simulink library "magField_lib"  (R2018b)
settings: Solver=VariableStepAuto  StartTime=0.0  StopTime=10.0  RelTol=1e-3
undefined symbols (not defined in the file or in its folder): Earth, fswParams, WGS84
libraries: aerolibtransform2 x3, aerolibgravity2 x1
settings Model: Creator=Kate  LastModifiedBy=devantormey

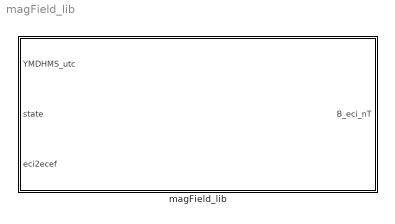
== system magField_lib ==
  magField_lib : Subsystem

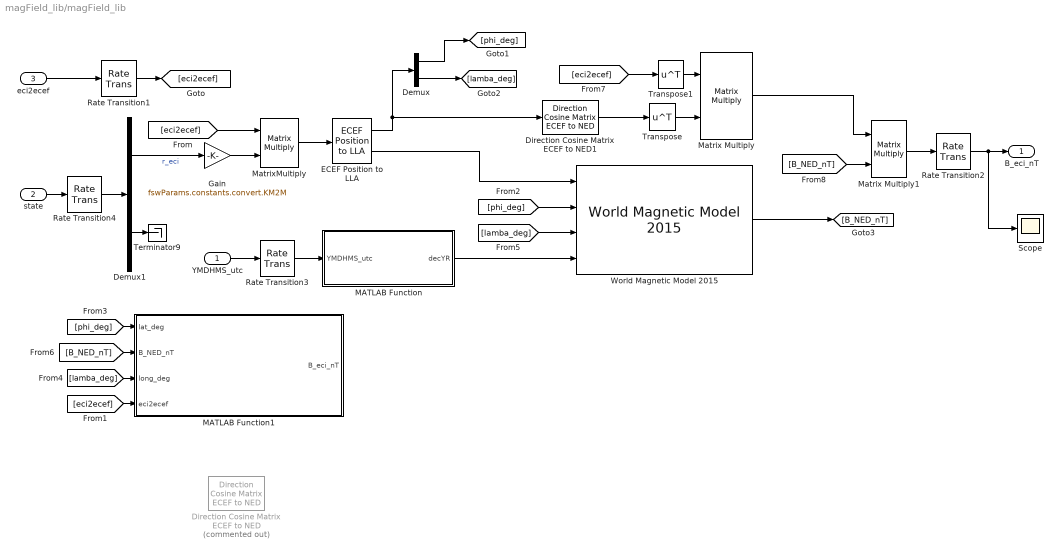
== system magField_lib/magField_lib ==
  YMDHMS_utc : Inport
  state : Inport  Port=2
  eci2ecef : Inport  Port=3
  Demux : Demux  Outputs=[1 1]
  Demux1 : Demux  Outputs=[3 10]
  Direction Cosine Matrix ECEF to NED : aerolibtransform2/Direction Cosine Matrix ECEF to NED  Commented=on
      settings: SourceProductName=Aerospace Blockset  SourceProductBaseCode=AE
  Direction Cosine Matrix ECEF to NED1 : aerolibtransform2/Direction Cosine Matrix ECEF to NED
      settings: SourceProductName=Aerospace Blockset  SourceProductBaseCode=AE
  ECEF Position to LLA : aerolibtransform2/ECEF Position to LLA  units=Metric (MKS)  ptype=Earth (WGS84)  F=1/298.257223563  R=6378137
      settings: SourceProductName=Aerospace Blockset  SourceProductBaseCode=AE
  Gain : Gain  Gain=fswParams.constants.convert.KM2M
  MATLAB Function : MATLAB Function  TreatAsAtomicUnit=on
  MATLAB Function1 : MATLAB Function  TreatAsAtomicUnit=on
  Matrix Multiply : Product  Multiplication=Matrix(*)
  Matrix Multiply1 : Product  Multiplication=Matrix(*)
  MatrixMultiply : Product  Multiplication=Matrix(*)
  Rate Transition1 : RateTransition  OutPortSampleTime=simParams.magField.sample_time_s
  Rate Transition2 : RateTransition
  Rate Transition3 : RateTransition  OutPortSampleTime=simParams.magField.sample_time_s
  Rate Transition4 : RateTransition  OutPortSampleTime=simParams.magField.sample_time_s
  Scope : Scope
  Terminator9 : Terminator
  Transpose : Math  Operator=transpose  SaturateOnIntegerOverflow=on
  Transpose1 : Math  Operator=transpose  SaturateOnIntegerOverflow=on
  World Magnetic Model 2015 : aerolibgravity2/World Magnetic Model 2015  units=Metric (MKS)  time_in=on  month=January  day=1  year=2015  action=Error  h_out=off  dec_out=off  inc_out=off  ti_out=off
      settings: SourceProductName=Aerospace Blockset  SourceProductBaseCode=AE
  B_eci_nT : Outport
  wires:
  Gain/1 -> MatrixMultiply/2
  Matrix Multiply1/1 -> Rate Transition2/1
  Rate Transition2/1 -> B_eci_nT/1, Scope/1
  [B_NED_nT] -> Matrix Multiply1/2
  Matrix Multiply/1 -> Matrix Multiply1/1
  Transpose/1 -> Matrix Multiply/2
  Transpose1/1 -> Matrix Multiply/1
  [eci2ecef] -> Transpose1/1
  Direction Cosine Matrix ECEF to NED1/1 -> Transpose/1
  Demux/2 -> [lamba_deg]
  Demux/1 -> [phi_deg]
  ECEF Position to LLA/1 -> Demux/1, Direction Cosine Matrix ECEF to NED1/1
  ECEF Position to LLA/2 -> World Magnetic Model 2015/1
  MatrixMultiply/1 -> ECEF Position to LLA/1
  MATLAB Function/1(decYR) -> World Magnetic Model 2015/4
  YMDHMS_utc/1 -> Rate Transition3/1
  Demux1/2 -> Terminator9/1
  Demux1/1 -> Gain/1  "r_eci"
  state/1 -> Rate Transition4/1
  eci2ecef/1 -> Rate Transition1/1
  [eci2ecef] -> MatrixMultiply/1
  [eci2ecef] -> MATLAB Function1/4(eci2ecef)
  Rate Transition4/1 -> Demux1/1
  Rate Transition1/1 -> [eci2ecef]
  Rate Transition3/1 -> MATLAB Function/1(YMDHMS_utc)
  [phi_deg] -> World Magnetic Model 2015/2
  [phi_deg] -> MATLAB Function1/1(lat_deg)
  [lamba_deg] -> World Magnetic Model 2015/3
  World Magnetic Model 2015/1 -> [B_NED_nT]
  [B_NED_nT] -> MATLAB Function1/2(B_NED_nT)
  [lamba_deg] -> MATLAB Function1/3(long_deg)

== matlab function magField_lib/MATLAB Function ==
  data: YMDHMS_utc input; decYR output
%function converts YMDHMS array to decimal years
function decYR = decyr(YMDHMS_utc)
year=YMDHMS_utc(1);
month=YMDHMS_utc(2);
day=YMDHMS_utc(3);
hour=YMDHMS_utc(4);
min=YMDHMS_utc(5);
sec=YMDHMS_utc(6);

janD=31;
marchD=31;
aprilD=30;
mayD=31;
juneD=30;
julyD=31; 
augD=31;
septD=30;
octD=31;
novD=30;



if mod(year,4)==0 %leap year
    daysT=366; %total days in year
    fedD=29;
else
    daysT=365.25;
    fedD=28;
end
    
if month == 1
    daysS= day; %days so far
elseif month ==2
    daysS=janD+day;
elseif month ==3
    daysS=janD+fedD+day;
elseif month==4
    daysS=janD+fedD+marchD+day;
elseif month==5
    daysS=janD+fedD+marchD+aprilD+day;
elseif month==6
    daysS=janD+fedD+marchD+aprilD+mayD+day;
elseif month==7
    daysS=janD+fedD+marchD+aprilD+mayD+juneD+day;
elseif month==8
    daysS=janD+fedD+marchD+aprilD+mayD+juneD+julyD+day;
elseif month==9
    daysS=janD+fedD+marchD+aprilD+mayD+juneD+julyD+augD+day;
elseif month==10
    daysS=janD+fedD+marchD+aprilD+mayD+juneD+julyD+augD+septD+day;
elseif month==11
    daysS=janD+fedD+marchD+aprilD+mayD+juneD+julyD+augD+septD+octD+day;
else %dec
    daysS=janD+fedD+marchD+aprilD+mayD+juneD+julyD+augD+septD+octD+novD+day;
end

%add time of day component
daysS=daysS+hour/24+min/1440+sec/86400;
decYR=year+daysS/daysT;
end

== matlab function magField_lib/MATLAB Function1 ==
  data: lat_deg input; B_NED_nT input; B_eci_nT output; long_deg input; eci2ecef input
function B_eci_nT = ned2eci(lat_deg,B_NED_nT,long_deg,eci2ecef)
%NED to ECEF
DCMef=zeros(3);
%source:https://www.mathworks.com/help/aeroblks/directioncosinematrixeceftoned.html
DCMef=[-sind(lat_deg)*cosd(long_deg) -sind(lat_deg)*sind(long_deg) cosd(lat_deg);...
    -sind(long_deg) cosd(long_deg) 0;...
    -cosd(lat_deg)*cosd(long_deg) -cosd(lat_deg)*sind(long_deg) -sind(lat_deg)];

B_ecef=transpose(DCMef)*B_NED_nT;

%ECEF to ECI using transformation matrix from time lib
B_eci_nT=transpose(eci2ecef)*B_ecef; %eci2ecef transformation matrix given by time_lib
end
